simulink model "ev_tms_v4_2022"  (R2023a)
settings: Solver=VariableStepAuto  StartTime=0.0  StopTime=inf  RelTol=1e-3  AbsTol=1e-3
model workspace: external: MATLAB File /Users/rossschrader/Documents/GitHub/RL_EV_TMS/blower_control/power_comparison/ev_tms_v4_params.m (data not in the file)
undefined symbols (not defined in the file): ac_onoff, battery_C1_LUT, battery_capacity_LUT, battery_cell_cp, battery_cell_mass, battery_Em_LUT, battery_N_cells, battery_Qe_init, battery_R0_LUT, battery_R1_LUT, battery_SOC_LUT, battery_T_init, battery_temperature_LUT, bulb, cabin_duct_area, cabin_T_init, chiller_area_primary, chiller_N_baffles, chiller_N_tubes, chiller_tube_D, chiller_tube_L, chiller_wall_conductivity, chiller_wall_thickness, compressor_rpm_LUT, condenser_air_area_flow, condenser_air_area_primary, condenser_W, condenser_wall_conductivity, condenser_wall_thickness, coolant_channel_D, coolant_pipe_D, coolant_T_init, coolant_tank_area, coolant_tank_volume, coolant_valve_D_ratio_max, coolant_valve_D_ratio_min, coolant_valve_displacement, coolant_valve_S_max, evaporator_air_area_flow, evaporator_air_area_primary, evaporator_P_target, evaporator_W, evaporator_wall_conductivity, evaporator_wall_thickness, outlet, pump_speed_max, radiator_air_area_flow, radiator_air_area_primary, radiator_W, radiator_wall_conductivity, radiator_wall_thickness, refrigerant_alpha_init, refrigerant_pipe_D, T_env, T_setpoint
libraries: fl_lib x221, nesl_utility x79, SimscapeFluids_lib x25, LiBatteryElements_lib x16, sdl_lib x3, slpidlib x2, simulink x1, rllib x1, autolibshared x1, SignalEditorBlockLib x1
(part 1 of 7)
CloseFcn:
  | try,close(h1_sscfluids_ev_thermal_management),end
  | clear h1_sscfluids_ev_thermal_management
  | 
  | clear tout simlog_sscfluids_ev_thermal_management
Description:
  | Electric Vehicle Thermal Management
settings Model: Creator=The MathWorks, Inc.  LastModifiedBy=rossschrader
settings SolverCC: AutoScaleAbsTol=off  MaxConsecutiveMinStep=4  ZeroCrossAlgorithm=Adaptive  AlgebraicLoopSolver=TrustRegion  MaxZcPerStep=1
settings DebuggingCC: MaxConsecutiveZCsMsg=none  IgnoredZcDiagnostic=none  UnconnectedInputMsg=warning  UnconnectedOutputMsg=warning  UnconnectedLineMsg=warning  SymbolicDimsDataTypeCodeGenerationDiagnostic=none
settings ModelReferenceCC: EnableRefExpFcnMdlSchedulingChecks=on
settings SFSimCC: CustomCodeUndefinedFunction=UseInterfaceOnly
settings RTWCC: DLArmComputeVersion=19.05
settings SimscapeCC: SimscapeLogType=all  SimscapeLogSimulationStatistics=on  SimscapeLogName=simlog_sscfluids_ev_thermal_management  SimscapeLogDataHistory=20000

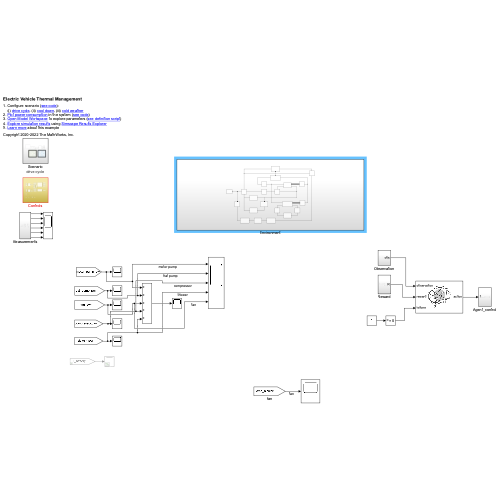
[thumbnail: Simulink's stored preview of the top-level diagram]
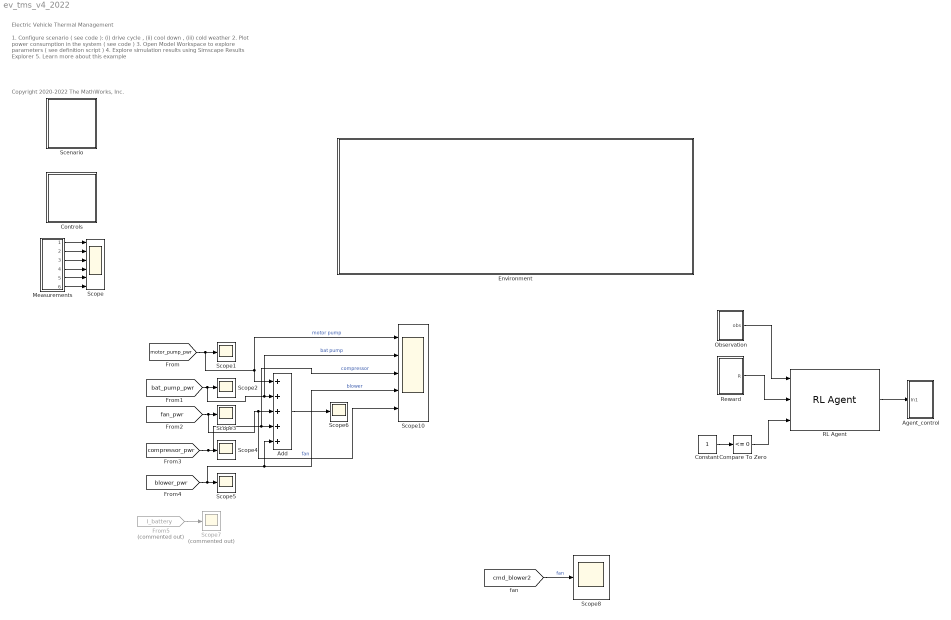
== system ev_tms_v4_2022 ==
  note: Electric Vehicle Thermal Management
  note: 1. Configure scenario ( see code ):
      | (i) drive cycle , (ii) cool down , (iii) cold weather
      | 2. Plot power consumption in the system ( see code )
      | 3. Open Model Workspace to explore parameters ( see definition script )
      | 4. Explore simulation results using Simscape Results Explorer
      | 5. Learn more about this example
  note: Copyright 2020-2022 The MathWorks, Inc.
  Add : Sum  Inputs=+++++
  Agent_control : Subsystem
  Compare To Zero : simulink/Logic and Bit Operations/Compare To Zero  relop=<=  OutDataTypeStr=boolean
  Constant : Constant
  Controls : Subsystem  Tag=PublishSubsystem
  Environment : Subsystem
  From5 : From  Commented=on  GotoTag=I_battery  TagVisibility=global
  Measurements : Subsystem
  Observation : Subsystem
  RL Agent : rllib/RL Agent  Agent=agentObj  ExternalActionAsInput=off  ProvideLastAction=off  ProvideCumRwd=off  TreatAsDirectFeedthrough=on  UseStrictObservationDataTypes=off
  Reward : Subsystem
  Scenario : Subsystem  Tag=drive cycle
      settings: AttributesFormatString=%<Tag>
  Scope : Scope  NumInputPorts=6
  Scope{1..6,8} (7 alike) : Scope
  Scope10 : Scope  NumInputPorts=5
  Scope7 : Scope  Commented=on
  wires:
  Measurements/1(Out1) -> Scope/1
  Measurements/2(Out2) -> Scope/2
  Measurements/3(Out3) -> Scope/3
  Measurements/4(Out4) -> Scope/4
  Measurements/5(Out5) -> Scope/5
  Measurements/6(Out6) -> Scope/6
  [bat_pump_pwr] -> Scope10/2, Add/2, Scope2/1  "bat pump"
  [fan_pwr] -> Scope10/5, Add/3, Scope3/1  "fan"
  [motor_pump_pwr] -> Scope10/1, Add/1, Scope1/1  "motor pump"
  [compressor_pwr] -> Scope10/3, Add/4, Scope4/1  "compressor"
  [blower_pwr] -> Scope10/4, Add/5, Scope5/1  "blower"
  Add/1 -> Scope6/1
  From5/1 -> Scope7/1
  Observation/1(obs) -> RL Agent/1
  Compare To Zero/1 -> RL Agent/3
  Constant/1 -> Compare To Zero/1
  Reward/1(R) -> RL Agent/2
  [cmd_blower2] -> Scope8/1  "fan"
  RL Agent/1 -> Agent_control/1(In1)

== system ev_tms_v4_2022/Agent_control ==
  In1 : Inport
  tag scope: cmd_blower2=global
  wires:
  In1/1 -> [cmd_blower2]

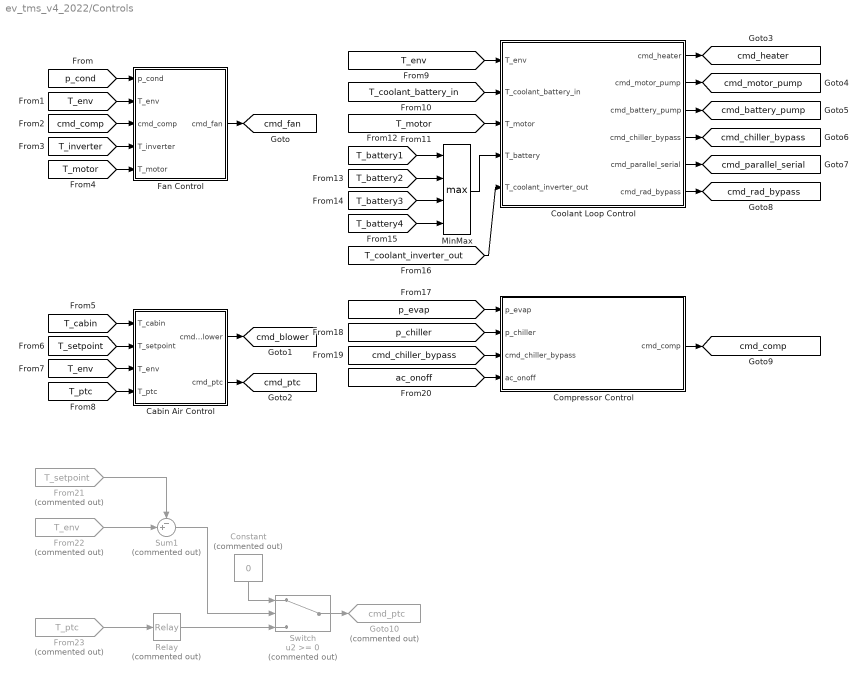
== system ev_tms_v4_2022/Controls ==
  Cabin Air Control : Subsystem
  Compressor Control : Subsystem
  Constant : Constant  Commented=on  Value=0
  Coolant Loop Control : Subsystem
  Fan Control : Subsystem
  From21 : From  Commented=on  GotoTag=T_setpoint  TagVisibility=global
  From22 : From  Commented=on  GotoTag=T_env  TagVisibility=global
  From23 : From  Commented=on  GotoTag=T_ptc  TagVisibility=global
  Goto10 : Goto  Commented=on  GotoTag=cmd_ptc  TagVisibility=global
  MinMax : MinMax  Function=max  Inputs=4
  Relay : Relay  Commented=on  OnSwitchValue=45  OffSwitchValue=35  OnOutputValue=0  OffOutputValue=1  ZeroCross=off
  Sum1 : Sum  Commented=on  Inputs=-+|
  Switch : Switch  Commented=on  SaturateOnIntegerOverflow=off  InputSameDT=off
  tag scope: cmd_battery_pump=global, cmd_blower=global, cmd_chiller_bypass=global, cmd_comp=global, cmd_fan=global, cmd_heater=global, cmd_motor_pump=global, cmd_parallel_serial=global, cmd_ptc=global, cmd_rad_bypass=global
  wires:
  [p_cond] -> Fan Control/1(p_cond)
  [T_env] -> Fan Control/2(T_env)
  [T_inverter] -> Fan Control/4(T_inverter)
  [T_motor] -> Fan Control/5(T_motor)
  [T_env] -> Coolant Loop Control/1(T_env)
  [T_coolant_battery_in] -> Coolant Loop Control/2(T_coolant_battery_in)
  Fan Control/1(cmd_fan) -> [cmd_fan]
  Coolant Loop Control/1(cmd_heater) -> [cmd_heater]
  Coolant Loop Control/2(cmd_motor_pump) -> [cmd_motor_pump]
  Coolant Loop Control/3(cmd_battery_pump) -> [cmd_battery_pump]
  [p_evap] -> Compressor Control/1(p_evap)
  [p_chiller] -> Compressor Control/2(p_chiller)
  [cmd_chiller_bypass] -> Compressor Control/3(cmd_chiller_bypass)
  [ac_onoff] -> Compressor Control/4(ac_onoff)
  Compressor Control/1(cmd_comp) -> [cmd_comp]
  Cabin Air Control/1(cmd_blower) -> [cmd_blower]
  Cabin Air Control/2(cmd_ptc) -> [cmd_ptc]
  Coolant Loop Control/4(cmd_chiller_bypass) -> [cmd_chiller_bypass]
  Coolant Loop Control/5(cmd_parallel_serial) -> [cmd_parallel_serial]
  Coolant Loop Control/6(cmd_rad_bypass) -> [cmd_rad_bypass]
  [T_motor] -> Coolant Loop Control/3(T_motor)
  [T_battery3] -> MinMax/3
  [T_battery4] -> MinMax/4
  [T_battery2] -> MinMax/2
  [T_battery1] -> MinMax/1
  [T_coolant_inverter_out] -> Coolant Loop Control/5(T_coolant_inverter_out)
  MinMax/1 -> Coolant Loop Control/4(T_battery)
  [cmd_comp] -> Fan Control/3(cmd_comp)
  [T_cabin] -> Cabin Air Control/1(T_cabin)
  [T_setpoint] -> Cabin Air Control/2(T_setpoint)
  [T_env] -> Cabin Air Control/3(T_env)
  [T_ptc] -> Cabin Air Control/4(T_ptc)
  Sum1/1 -> Switch/2
  From23/1 -> Relay/1
  Constant/1 -> Switch/1
  From21/1 -> Sum1/1
  Relay/1 -> Switch/3
  From22/1 -> Sum1/2
  Switch/1 -> Goto10/1

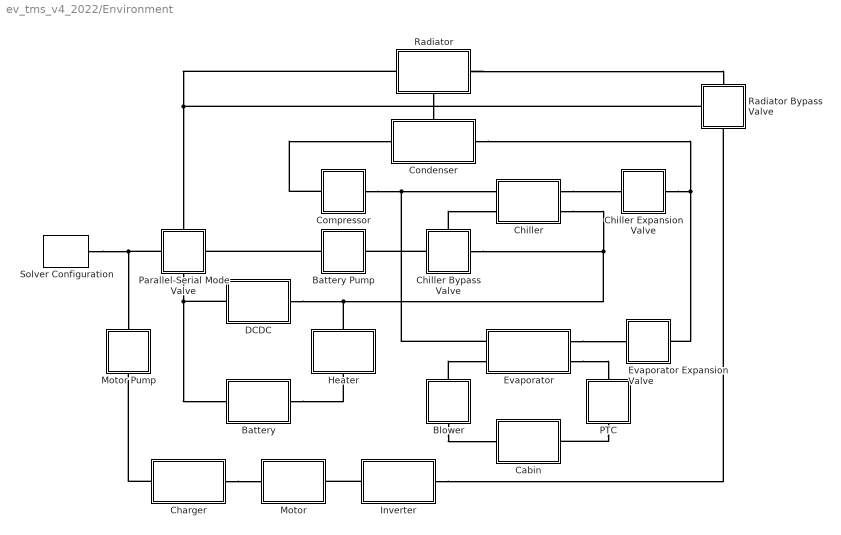
== system ev_tms_v4_2022/Environment ==
  Battery : Subsystem  Tag=PublishSubsystem
      mask Display: disp(get_param(gcb, 'Name'))
  Battery Pump : Subsystem  Tag=PublishSubsystem
      mask Display:
      | plot(100*cos(linspace(0, 2*pi, 500)), 100*sin(linspace(0, 2*pi, 500)))
      | patch([100 55 55 100]-1, [0 24 -24 0], [0 0 0])
  Blower : Subsystem  Tag=PublishSubsystem
      settings: PortSchema="{\"entries\":[{\"content\":{\"sides\":[{\"content\":{\"connectorIds\":[]},\"type\":\"ConnectorPlacement.EquallySpacedRectSide\",\"uuid\":\"e68f4e4f-d2a0-4f21-a3dd-a8ccea0ce87c\"},{\"content\":{\"connectorIds\":[],\"side\":\"RIGHT\"},\"type\":\"ConnectorPlacement.EquallySpacedRectSide\",\"uuid\":\"01f15736-e6d7-4b17-9e84-cef8e8356dfe\"},{\"content\":{\"connectorIds\":[\"LConn1\"],\"side\":\"TOP\"},\"type\":\"ConnectorPlacement.EquallySpacedRectSide\",\"uuid\":\"cb1790c7-7993-46e4-a971-f0b801f1d2ca\"},{\"content\":{\"connectorIds\":[\"RConn1\"],\"side\":\"BOTTOM\"},\"type\":\"ConnectorPlacement.EquallySpacedRectSide\",\"uuid\":\"4227c4aa-9146-4cfe-9198-d14a991805e7\"},{\"content\":{\"connectorIds\":[],\"side\":\"HIDDEN\"},\"type\":\"ConnectorPlacement.EquallySpacedRectSide\",\"uuid\":\"e2e3575c-3b20-453d-a897-62a34bc693b5\"}]},\"type\":\"ConnectorPlacement.EquallySpacedConnector\",\"uuid\":\"0a7b2bb7-4c38-48ec-bfc1-fef0f38ff266\"}],\"packageUris\":[\"http://schema.mathworks.com/mf0/Connector/R2020b\"],\"version\":\"1.0\"}"
      mask Display:
      | plot(100*cos(linspace(0, 2*pi, 500)), 100*sin(linspace(0, 2*pi, 500)))
      | plot([28 80], [96 -60])
      | plot([-28 -80], [96 -60])
      | patch(-50*sin(3*linspace(0, pi, 500)).*cos(linspace(0, pi, 500)), -50*sin(3*linspace(0, pi, 500)).*sin(linspace(0, pi, 500)), [0 0 0])
  Cabin : Subsystem  Tag=PublishSubsystem
      mask Display: disp(get_param(gcb, 'Name'))
  Charger : Subsystem  Tag=PublishSubsystem
      mask Display: disp(get_param(gcb, 'Name'))
  Chiller : Subsystem  Tag=PublishSubsystem
      mask Display: disp(get_param(gcb, 'Name'))
  Chiller Bypass Valve : Subsystem  Tag=PublishSubsystem
      settings: PortSchema="{\"entries\":[{\"content\":{\"sides\":[{\"content\":{\"connectorIds\":[\"LConn1\"]},\"type\":\"ConnectorPlacement.EquallySpacedRectSide\",\"uuid\":\"c08eba77-a229-49ef-96a6-5debb89bda6a\"},{\"content\":{\"connectorIds\":[\"RConn1\"],\"side\":\"RIGHT\"},\"type\":\"ConnectorPlacement.EquallySpacedRectSide\",\"uuid\":\"bf1c3c92-2d76-498b-aaec-772d925127f1\"},{\"content\":{\"connectorIds\":[\"LConn2\"],\"side\":\"TOP\"},\"type\":\"ConnectorPlacement.EquallySpacedRectSide\",\"uuid\":\"93e37f17-addf-4d5b-9a57-68c15f6f3e9e\"},{\"content\":{\"connectorIds\":[],\"side\":\"HIDDEN\"},\"type\":\"ConnectorPlacement.EquallySpacedRectSide\",\"uuid\":\"04fa26e7-4471-4f20-81b8-29848726d0cd\"}]},\"type\":\"ConnectorPlacement.EquallySpacedConnector\",\"uuid\":\"712c9662-e870-49a5-b0e3-dc86b008bacd\"}],\"packageUris\":[\"http://schema.mathworks.com/mf0/Connector/R2020b\"],\"version\":\"1.0\"}"
      mask Display:
      | color('white')
      | plot(100, 100)
      | plot(-100, -100)
      | color('black')
      | 
      | plot([0 -100 -100 0], [0 50 -50 0])
      | plot([0 100 100 0], [0 50 -50 0])
      | plot([0 50 -50 0], [0 100 100 0])
  Chiller Expansion Valve : Subsystem  Tag=PublishSubsystem
      mask Display:
      | color('white')
      | plot(100, 100)
      | plot(-100, -100)
      | color('black')
      | 
      | plot([0 -100 -100 0], [0 50 -50 0])
      | plot([0 100 100 0], [0 50 -50 0])
  Compressor : Subsystem  Tag=PublishSubsystem
      mask Display:
      | plot(100*cos(linspace(0, 2*pi, 500)), 100*sin(linspace(0, 2*pi, 500)))
      | plot([-96 60], [28 80])
      | plot([-96 60], [-28 -80])
  Condenser : Subsystem  Tag=PublishSubsystem
      settings: PortSchema="{\"entries\":[{\"content\":{\"sides\":[{\"content\":{\"connectorIds\":[\"LConn1\"]},\"type\":\"ConnectorPlacement.EquallySpacedRectSide\",\"uuid\":\"1c8aa983-a374-4f1b-b303-31d972477bc1\"},{\"content\":{\"connectorIds\":[\"RConn1\"],\"side\":\"RIGHT\"},\"type\":\"ConnectorPlacement.EquallySpacedRectSide\",\"uuid\":\"9470a7c4-8d01-4f33-b281-130c1633b9af\"},{\"content\":{\"connectorIds\":[\"LConn2\"],\"side\":\"TOP\"},\"type\":\"ConnectorPlacement.EquallySpacedRectSide\",\"uuid\":\"521bcd61-502e-4408-add3-862bd83fd72a\"},{\"content\":{\"connectorIds\":[],\"side\":\"HIDDEN\"},\"type\":\"ConnectorPlacement.EquallySpacedRectSide\",\"uuid\":\"1fd51896-89cd-4b86-8982-5d9c8888072c\"}]},\"type\":\"ConnectorPlacement.EquallySpacedConnector\",\"uuid\":\"d9db812f-15c4-4875-aa5b-4de8fb002b03\"}],\"packageUris\":[\"http://schema.mathworks.com/mf0/Connector/R2020b\"],\"version\":\"1.0\"}"
      mask Display: disp(get_param(gcb, 'Name'))
  DCDC : Subsystem  Tag=PublishSubsystem
      mask Display: disp(get_param(gcb, 'Name'))
  Evaporator : Subsystem  Tag=PublishSubsystem
      mask Display: disp(get_param(gcb, 'Name'))
  Evaporator Expansion Valve : Subsystem  Tag=PublishSubsystem
      mask Display:
      | color('white')
      | plot(100, 100)
      | plot(-100, -100)
      | color('black')
      | 
      | plot([0 -100 -100 0], [0 50 -50 0])
      | plot([0 100 100 0], [0 50 -50 0])
  Heater : Subsystem  Tag=PublishSubsystem
      settings: PortSchema="{\"entries\":[{\"content\":{\"sides\":[{\"content\":{\"connectorIds\":[]},\"type\":\"ConnectorPlacement.EquallySpacedRectSide\",\"uuid\":\"e68f4e4f-d2a0-4f21-a3dd-a8ccea0ce87c\"},{\"content\":{\"connectorIds\":[],\"side\":\"RIGHT\"},\"type\":\"ConnectorPlacement.EquallySpacedRectSide\",\"uuid\":\"01f15736-e6d7-4b17-9e84-cef8e8356dfe\"},{\"content\":{\"connectorIds\":[\"LConn1\"],\"side\":\"TOP\"},\"type\":\"ConnectorPlacement.EquallySpacedRectSide\",\"uuid\":\"cb1790c7-7993-46e4-a971-f0b801f1d2ca\"},{\"content\":{\"connectorIds\":[\"RConn1\"],\"side\":\"BOTTOM\"},\"type\":\"ConnectorPlacement.EquallySpacedRectSide\",\"uuid\":\"c273a181-4a30-4811-b574-293af963aa70\"},{\"content\":{\"connectorIds\":[],\"side\":\"HIDDEN\"},\"type\":\"ConnectorPlacement.EquallySpacedRectSide\",\"uuid\":\"e2e3575c-3b20-453d-a897-62a34bc693b5\"}]},\"type\":\"ConnectorPlacement.EquallySpacedConnector\",\"uuid\":\"0a7b2bb7-4c38-48ec-bfc1-fef0f38ff266\"}],\"packageUris\":[\"http://schema.mathworks.com/mf0/Connector/R2020b\"],\"version\":\"1.0\"}"
      mask Display: disp(get_param(gcb, 'Name'))
  Inverter : Subsystem  Tag=PublishSubsystem
      mask Display: disp(get_param(gcb, 'Name'))
  Motor : Subsystem  Tag=PublishSubsystem
      mask Display: disp(get_param(gcb, 'Name'))
  Motor Pump : Subsystem  Tag=PublishSubsystem
      settings: PortSchema="{\"entries\":[{\"content\":{\"sides\":[{\"content\":{\"connectorIds\":[]},\"type\":\"ConnectorPlacement.EquallySpacedRectSide\",\"uuid\":\"e68f4e4f-d2a0-4f21-a3dd-a8ccea0ce87c\"},{\"content\":{\"connectorIds\":[],\"side\":\"RIGHT\"},\"type\":\"ConnectorPlacement.EquallySpacedRectSide\",\"uuid\":\"01f15736-e6d7-4b17-9e84-cef8e8356dfe\"},{\"content\":{\"connectorIds\":[\"LConn1\"],\"side\":\"TOP\"},\"type\":\"ConnectorPlacement.EquallySpacedRectSide\",\"uuid\":\"cb1790c7-7993-46e4-a971-f0b801f1d2ca\"},{\"content\":{\"connectorIds\":[\"RConn1\"],\"side\":\"BOTTOM\"},\"type\":\"ConnectorPlacement.EquallySpacedRectSide\",\"uuid\":\"8246d38e-a008-4f4a-9c4c-9e03a2298f65\"},{\"content\":{\"connectorIds\":[],\"side\":\"HIDDEN\"},\"type\":\"ConnectorPlacement.EquallySpacedRectSide\",\"uuid\":\"e2e3575c-3b20-453d-a897-62a34bc693b5\"}]},\"type\":\"ConnectorPlacement.EquallySpacedConnector\",\"uuid\":\"0a7b2bb7-4c38-48ec-bfc1-fef0f38ff266\"}],\"packageUris\":[\"http://schema.mathworks.com/mf0/Connector/R2020b\"],\"version\":\"1.0\"}"
      mask Display:
      | plot(100*cos(linspace(0, 2*pi, 500)), 100*sin(linspace(0, 2*pi, 500)))
      | patch([0 24 -24 0], [-100 -55 -55 -100]+1, [0 0 0])
  PTC : Subsystem  Tag=PublishSubsystem
      settings: PortSchema="{\"entries\":[{\"content\":{\"sides\":[{\"content\":{\"connectorIds\":[]},\"type\":\"ConnectorPlacement.EquallySpacedRectSide\",\"uuid\":\"e68f4e4f-d2a0-4f21-a3dd-a8ccea0ce87c\"},{\"content\":{\"connectorIds\":[],\"side\":\"RIGHT\"},\"type\":\"ConnectorPlacement.EquallySpacedRectSide\",\"uuid\":\"01f15736-e6d7-4b17-9e84-cef8e8356dfe\"},{\"content\":{\"connectorIds\":[\"LConn1\"],\"side\":\"TOP\"},\"type\":\"ConnectorPlacement.EquallySpacedRectSide\",\"uuid\":\"cb1790c7-7993-46e4-a971-f0b801f1d2ca\"},{\"content\":{\"connectorIds\":[\"RConn1\"],\"side\":\"BOTTOM\"},\"type\":\"ConnectorPlacement.EquallySpacedRectSide\",\"uuid\":\"8429c419-0ca8-47a9-96c7-e8d1ee01deb6\"},{\"content\":{\"connectorIds\":[],\"side\":\"HIDDEN\"},\"type\":\"ConnectorPlacement.EquallySpacedRectSide\",\"uuid\":\"e2e3575c-3b20-453d-a897-62a34bc693b5\"}]},\"type\":\"ConnectorPlacement.EquallySpacedConnector\",\"uuid\":\"0a7b2bb7-4c38-48ec-bfc1-fef0f38ff266\"}],\"packageUris\":[\"http://schema.mathworks.com/mf0/Connector/R2020b\"],\"version\":\"1.0\"}"
      mask Display: disp(get_param(gcb, 'Name'))
  Parallel-Serial Mode Valve : Subsystem  Tag=PublishSubsystem
      settings: PortSchema="{\"entries\":[{\"content\":{\"sides\":[{\"content\":{\"connectorIds\":[\"LConn1\"]},\"type\":\"ConnectorPlacement.EquallySpacedRectSide\",\"uuid\":\"769cdae0-dc58-4cfd-92d9-ac32508c6b10\"},{\"content\":{\"connectorIds\":[\"RConn1\"],\"side\":\"RIGHT\"},\"type\":\"ConnectorPlacement.EquallySpacedRectSide\",\"uuid\":\"df63fb06-baf4-4717-a479-9d23ab47f4aa\"},{\"content\":{\"connectorIds\":[\"LConn2\"],\"side\":\"TOP\"},\"type\":\"ConnectorPlacement.EquallySpacedRectSide\",\"uuid\":\"82fb49eb-ec90-48c3-a5a6-67a52560ca4a\"},{\"content\":{\"connectorIds\":[\"RConn2\"],\"side\":\"BOTTOM\"},\"type\":\"ConnectorPlacement.EquallySpacedRectSide\",\"uuid\":\"ab7ba56f-69df-4d32-95cc-f479df491f70\"},{\"content\":{\"connectorIds\":[],\"side\":\"HIDDEN\"},\"type\":\"ConnectorPlacement.EquallySpacedRectSide\",\"uuid\":\"14514675-c4ca-4da0-9eea-4f242d50599f\"}]},\"type\":\"ConnectorPlacement.EquallySpacedConnector\",\"uuid\":\"38d91077-2bde-4773-8967-83aa2a8f4957\"}],\"packageUris\":[\"http://schema.mathworks.com/mf0/Connector/R2020b\"],\"version\":\"1.0\"}"
      mask Display:
      | color('white')
      | plot(100, 100)
      | plot(-100, -100)
      | color('black')
      | 
      | plot([0 -100 -100 0], [0 50 -50 0])
      | plot([0 100 100 0], [0 50 -50 0])
      | plot([0 50 -50 0], [0 100 100 0])
      | plot([0 50 -50 0], [0 -100 -100 0])
  Radiator : Subsystem  Tag=PublishSubsystem
      settings: PortSchema="{\"entries\":[{\"content\":{\"sides\":[{\"content\":{\"connectorIds\":[\"LConn1\"]},\"type\":\"ConnectorPlacement.EquallySpacedRectSide\",\"uuid\":\"c41edd26-4d41-4ef4-bf36-0d7d2de0fe84\"},{\"content\":{\"connectorIds\":[\"RConn1\"],\"side\":\"RIGHT\"},\"type\":\"ConnectorPlacement.EquallySpacedRectSide\",\"uuid\":\"d74127b5-b0c6-43ff-8d29-bbb0795bdd4e\"},{\"content\":{\"connectorIds\":[],\"side\":\"TOP\"},\"type\":\"ConnectorPlacement.EquallySpacedRectSide\",\"uuid\":\"8924700c-666b-431d-af64-838d19a43fe5\"},{\"content\":{\"connectorIds\":[\"RConn2\"],\"side\":\"BOTTOM\"},\"type\":\"ConnectorPlacement.EquallySpacedRectSide\",\"uuid\":\"806c213f-7f35-4ea6-bb4b-65a47516f414\"},{\"content\":{\"connectorIds\":[],\"side\":\"HIDDEN\"},\"type\":\"ConnectorPlacement.EquallySpacedRectSide\",\"uuid\":\"7380b933-a71f-43b9-ae5a-a995a710e36b\"}]},\"type\":\"ConnectorPlacement.EquallySpacedConnector\",\"uuid\":\"07da1dfa-e3e5-4e48-89d5-0544451f2413\"}],\"packageUris\":[\"http://schema.mathworks.com/mf0/Connector/R2020b\"],\"version\":\"1.0\"}"
      mask Display: disp(get_param(gcb, 'Name'))
  Radiator Bypass Valve : Subsystem  Tag=PublishSubsystem
      settings: PortSchema="{\"entries\":[{\"content\":{\"sides\":[{\"content\":{\"connectorIds\":[\"LConn1\"]},\"type\":\"ConnectorPlacement.EquallySpacedRectSide\",\"uuid\":\"1991dfbd-c304-4807-b100-246bfad34882\"},{\"content\":{\"connectorIds\":[],\"side\":\"RIGHT\"},\"type\":\"ConnectorPlacement.EquallySpacedRectSide\",\"uuid\":\"8dd83d3e-3811-40e7-af6b-04929d024ef5\"},{\"content\":{\"connectorIds\":[\"LConn2\"],\"side\":\"TOP\"},\"type\":\"ConnectorPlacement.EquallySpacedRectSide\",\"uuid\":\"fac05c8b-fd4c-4caf-8f39-67a22531bfff\"},{\"content\":{\"connectorIds\":[\"RConn1\"],\"side\":\"BOTTOM\"},\"type\":\"ConnectorPlacement.EquallySpacedRectSide\",\"uuid\":\"fc2a2150-414c-4914-a21f-f7fbe52b92e3\"},{\"content\":{\"connectorIds\":[],\"side\":\"HIDDEN\"},\"type\":\"ConnectorPlacement.EquallySpacedRectSide\",\"uuid\":\"26904e98-8b18-4b4d-8057-298167e4cabd\"}]},\"type\":\"ConnectorPlacement.EquallySpacedConnector\",\"uuid\":\"c94d3059-f972-4f57-b434-9a5f1e7a2893\"}],\"packageUris\":[\"http://schema.mathworks.com/mf0/Connector/R2020b\"],\"version\":\"1.0\"}"
      mask Display:
      | color('white')
      | plot(100, 100)
      | plot(-100, -100)
      | color('black')
      | 
      | plot([0 -100 -100 0], [0 50 -50 0])
      | plot([0 50 -50 0], [0 100 100 0])
      | plot([0 50 -50 0], [0 -100 -100 0])
  Solver Configuration : nesl_utility/Solver Configuration  PhysicalDomain=network_engine_domain  SubClassName=solver  LeftPortType=input  RightPortType=generic  Tones=[]  Harmonics=[]  SimulateNoise=off  Profile=off  UseLocalSampling=off  EnableSwitchedLinearOptims=on  FrequencyDomain=off  UseCCode=off  RelTol=0.001  AbsTol=1e-06  MinStep=1e-09  ToWorkspace=off  RevertToSquareIcSolve=off  NumHomotopyIterations=100  PhasorMode=off  PhasorModeNumHarmonics=1  ConsistencySolver=NEWTON_XTOL_AFTER_FTOL  IndexReductionMethod=DerivativeReplacement  DoDC=off  ResidualTolerance=1e-09  ConsistencyTolSource=GLOBAL  ConsistencyAbsTol=0.001  ConsistencyRelTol=0.001  ConsistencyTolFactor=0.001  UseLocalSolver=off  LocalSolverChoice=NE_BACKWARD_EULER_ADVANCER  ResolveIndetEquations=on  FunctionEvalNumThread=1  LocalSolverSampleTime=0.001  DoFixedCost=off  MaxNonlinIter=3  MaxModeIter=2  ComputeImpulses=off  ImpulseIterations=2  LinearAlgebra=auto  LinearAlgebraNumThread=0  EquationFormulation=NE_TIME_EF  DelaysMemoryBudget=1024  AutomaticFiltering=on  FilteringTimeConstant=0.001  PartitionStorageMethod=AS_NEEDED  PartitionMemoryBudget=1024  PartitionMethod=ROBUST
  connections:
  Inverter/RConn1 -- Radiator Bypass Valve/RConn1
  Evaporator/RConn2 -- PTC/LConn1
  Parallel-Serial Mode Valve/LConn1 -- Solver Configuration/RConn1 -- Motor Pump/LConn1
  PTC/RConn1 -- Cabin/RConn1
  Blower/LConn1 -- Evaporator/LConn2
  Blower/RConn1 -- Cabin/LConn1
  Condenser/RConn1 -- Chiller Expansion Valve/RConn1 -- Evaporator Expansion Valve/RConn1
  Radiator/RConn1 -- Radiator Bypass Valve/LConn2
  Evaporator/RConn1 -- Evaporator Expansion Valve/LConn1
  Battery/RConn1 -- Heater/RConn1
  Chiller Bypass Valve/LConn1 -- Battery Pump/RConn1
  Radiator/RConn2 -- Condenser/LConn2
  Radiator/LConn1 -- Radiator Bypass Valve/LConn1 -- Parallel-Serial Mode Valve/LConn2
  Compressor/RConn1 -- Evaporator/LConn1 -- Chiller/LConn1
  Parallel-Serial Mode Valve/RConn2 -- DCDC/LConn1 -- Battery/LConn1
  Charger/RConn1 -- Motor/LConn1
  Chiller/RConn2 -- DCDC/RConn1 -- Heater/LConn1 -- Chiller Bypass Valve/RConn1
  Charger/LConn1 -- Motor Pump/RConn1
  Battery Pump/LConn1 -- Parallel-Serial Mode Valve/RConn1
  Chiller/RConn1 -- Chiller Expansion Valve/LConn1
  Chiller Bypass Valve/LConn2 -- Chiller/LConn2
  Compressor/LConn1 -- Condenser/LConn1
  Inverter/LConn1 -- Motor/RConn1

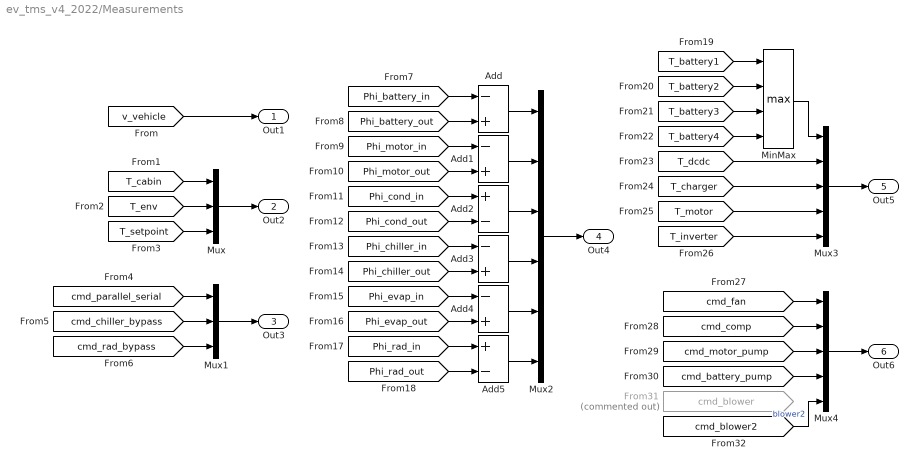
== system ev_tms_v4_2022/Measurements ==
  Add{,1,3..4} (4 alike) : Sum  Inputs=-+
  Add2 : Sum  Inputs=+-
  Add5 : Sum  Inputs=+-
  From31 : From  Commented=on  GotoTag=cmd_blower  TagVisibility=global
  MinMax : MinMax  Function=max  Inputs=4
  Mux : Mux  Inputs=3
  Mux1 : Mux  Inputs=3
  Mux2 : Mux  Inputs=6
  Mux3 : Mux  Inputs=5
  Mux4 : Mux  Inputs=5
  Out1 : Outport
  Out2 : Outport  Port=2
  Out3 : Outport  Port=3
  Out4 : Outport  Port=4
  Out5 : Outport  Port=5
  Out6 : Outport  Port=6
  wires:
  [v_vehicle] -> Out1/1
  [T_cabin] -> Mux/1
  [T_env] -> Mux/2
  [T_setpoint] -> Mux/3
  Mux/1 -> Out2/1
  [cmd_parallel_serial] -> Mux1/1
  [cmd_chiller_bypass] -> Mux1/2
  [cmd_rad_bypass] -> Mux1/3
  Mux1/1 -> Out3/1
  [Phi_battery_in] -> Add/1
  [Phi_battery_out] -> Add/2
  [Phi_motor_in] -> Add1/1
  [Phi_motor_out] -> Add1/2
  [Phi_cond_in] -> Add2/1
  [Phi_cond_out] -> Add2/2
  [Phi_chiller_in] -> Add3/1
  [Phi_chiller_out] -> Add3/2
  [Phi_evap_in] -> Add4/1
  [Phi_evap_out] -> Add4/2
  [Phi_rad_in] -> Add5/1
  [Phi_rad_out] -> Add5/2
  Add/1 -> Mux2/1
  Add1/1 -> Mux2/2
  Add2/1 -> Mux2/3
  Add3/1 -> Mux2/4
  Add4/1 -> Mux2/5
  Add5/1 -> Mux2/6
  Mux2/1 -> Out4/1
  [T_battery1] -> MinMax/1
  [T_battery2] -> MinMax/2
  [T_battery3] -> MinMax/3
  [T_battery4] -> MinMax/4
  [T_dcdc] -> Mux3/2
  [T_charger] -> Mux3/3
  [T_motor] -> Mux3/4
  [T_inverter] -> Mux3/5
  MinMax/1 -> Mux3/1
  Mux3/1 -> Out5/1
  [cmd_fan] -> Mux4/1
  [cmd_comp] -> Mux4/2
  [cmd_motor_pump] -> Mux4/3
  [cmd_battery_pump] -> Mux4/4
  Mux4/1 -> Out6/1
  [cmd_blower2] -> Mux4/5  "blower2"

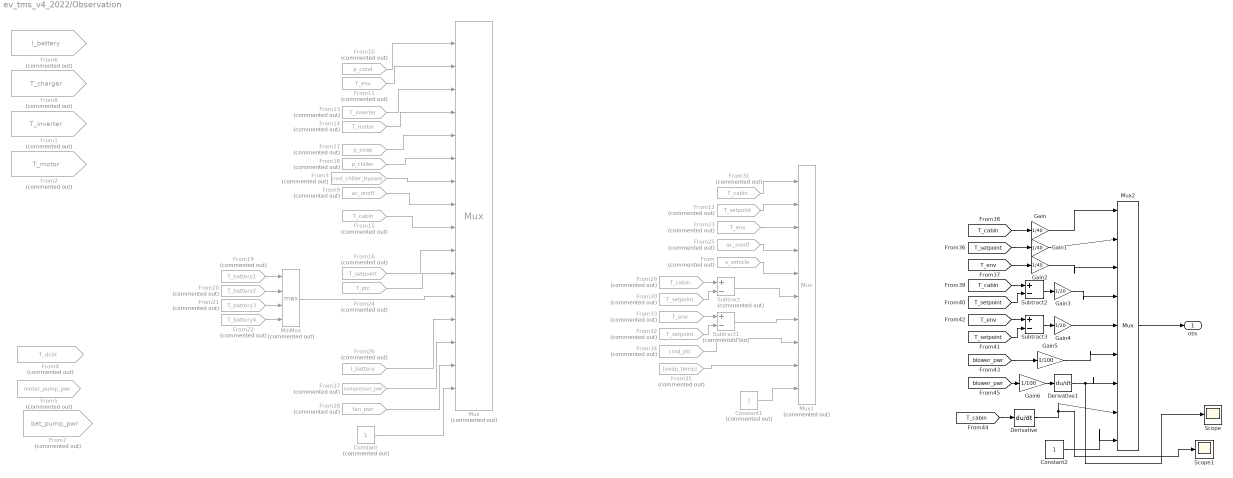
== system ev_tms_v4_2022/Observation ==
  Constant : Constant  Commented=on
  Constant1 : Constant  Commented=on
  Constant2 : Constant
  Derivative : Derivative
  Derivative1 : Derivative
  From : From  Commented=on  GotoTag=v_vehicle  TagVisibility=global
  From1 : From  Commented=on  GotoTag=T_inverter  TagVisibility=global
  From10 : From  Commented=on  GotoTag=p_cond  TagVisibility=global
  From11 : From  Commented=on  GotoTag=T_env  TagVisibility=global
  From{12,16,30,32} (4 alike) : From  Commented=on  GotoTag=T_setpoint  TagVisibility=global
  From13 : From  Commented=on  GotoTag=T_inverter  TagVisibility=global
  From14 : From  Commented=on  GotoTag=T_motor  TagVisibility=global
  From15 : From  Commented=on  GotoTag=T_cabin  TagVisibility=global
  From17 : From  Commented=on  GotoTag=p_evap  TagVisibility=global
  From18 : From  Commented=on  GotoTag=p_chiller  TagVisibility=global
  From19 : From  Commented=on  GotoTag=T_battery1  TagVisibility=global
  From2 : From  Commented=on  GotoTag=T_motor  TagVisibility=global
  From20 : From  Commented=on  GotoTag=T_battery2  TagVisibility=global
  From21 : From  Commented=on  GotoTag=T_battery3  TagVisibility=global
  From22 : From  Commented=on  GotoTag=T_battery4  TagVisibility=global
  From23 : From  Commented=on  GotoTag=T_env  TagVisibility=global
  From24 : From  Commented=on  GotoTag=T_ptc  TagVisibility=global
  From25 : From  Commented=on  GotoTag=ac_onoff  TagVisibility=global
  From26 : From  Commented=on  GotoTag=I_battery  TagVisibility=global
  From27 : From  Commented=on  GotoTag=compressor_pwr  TagVisibility=global
  From28 : From  Commented=on  GotoTag=fan_pwr  TagVisibility=global
  From29 : From  Commented=on  GotoTag=T_cabin  TagVisibility=global
  From3 : From  Commented=on  GotoTag=cmd_chiller_bypass  TagVisibility=global
  From31 : From  Commented=on  GotoTag=T_cabin  TagVisibility=global
  From33 : From  Commented=on  GotoTag=T_env  TagVisibility=global
  From34 : From  Commented=on  GotoTag=cmd_ptc  TagVisibility=global
  From35 : From  Commented=on  GotoTag=evap_temp  TagVisibility=global
  From4 : From  Commented=on  GotoTag=T_dcdc  TagVisibility=global
  From5 : From  Commented=on  GotoTag=motor_pump_pwr  TagVisibility=global
  From6 : From  Commented=on  GotoTag=I_battery  TagVisibility=global
  From7 : From  Commented=on  GotoTag=bat_pump_pwr  TagVisibility=global
  From8 : From  Commented=on  GotoTag=T_charger  TagVisibility=global
  From9 : From  Commented=on  GotoTag=ac_onoff  TagVisibility=global
  Gain : Gain  Gain=1/40
  Gain1 : Gain  Gain=1/40
  Gain2 : Gain  Gain=1/40
  Gain3 : Gain  Gain=1/20
  Gain4 : Gain  Gain=1/20
  Gain5 : Gain  Gain=1/100
  Gain6 : Gain  Gain=1/100
  MinMax : MinMax  Commented=on  Function=max  Inputs=4
  Mux : Mux  Commented=on  Inputs=16
  Mux1 : Mux  Commented=on  Inputs=10
  Mux2 : Mux  Inputs=9
  Scope : Scope
  Scope1 : Scope
  Subtract : Sum  Commented=on  Inputs=+-
  Subtract1 : Sum  Commented=on  Inputs=+-
  Subtract2 : Sum  Inputs=+-
  Subtract3 : Sum  Inputs=+-
  obs : Outport
  wires:
  From19/1 -> MinMax/1
  From20/1 -> MinMax/2
  From22/1 -> MinMax/4
  From21/1 -> MinMax/3
  MinMax/1 -> Mux/12
  From10/1 -> Mux/1
  From11/1 -> Mux/2
  From13/1 -> Mux/3
  From14/1 -> Mux/4
  From17/1 -> Mux/5
  From18/1 -> Mux/6
  From3/1 -> Mux/7
  From9/1 -> Mux/8
  From15/1 -> Mux/9
  From16/1 -> Mux/10
  From24/1 -> Mux/11
  From26/1 -> Mux/13
  From27/1 -> Mux/14
  From28/1 -> Mux/15
  Constant/1 -> Mux/16
  From31/1 -> Mux1/1
  From12/1 -> Mux1/2
  From23/1 -> Mux1/3
  From25/1 -> Mux1/4
  From/1 -> Mux1/5
  Constant1/1 -> Mux1/10
  From29/1 -> Subtract/1
  From30/1 -> Subtract/2
  Subtract/1 -> Mux1/6
  From33/1 -> Subtract1/1
  From32/1 -> Subtract1/2
  Subtract1/1 -> Mux1/7
  From34/1 -> Mux1/8
  From35/1 -> Mux1/9
  [T_cabin] -> Subtract2/1
  [T_env] -> Subtract3/1
  [T_setpoint] -> Subtract2/2
  [T_setpoint] -> Subtract3/2
  Mux2/1 -> obs/1
  [T_cabin] -> Gain/1
  [T_setpoint] -> Gain1/1
  [T_env] -> Gain2/1
  Subtract2/1 -> Gain3/1
  Subtract3/1 -> Gain4/1
  [blower_pwr] -> Gain5/1
  Gain/1 -> Mux2/1
  Gain1/1 -> Mux2/2
  Gain2/1 -> Mux2/3
  Gain3/1 -> Mux2/4
  Gain4/1 -> Mux2/5
  Gain5/1 -> Mux2/6
  Constant2/1 -> Mux2/9
  [T_cabin] -> Derivative/1
  Derivative/1 -> Scope1/1, Mux2/8
  [blower_pwr] -> Gain6/1
  Gain6/1 -> Derivative1/1
  Derivative1/1 -> Scope/1, Mux2/7

== system ev_tms_v4_2022/Reward ==
  Add : Sum
  Power Reward : Subsystem
  Scope : Scope  NumInputPorts=2
  Temp Reward : Subsystem
  R : Outport
  wires:
  Add/1 -> R/1
  Power Reward/1(Power) -> Scope/1, Add/1
  Temp Reward/1(Temp) -> Scope/2, Add/2

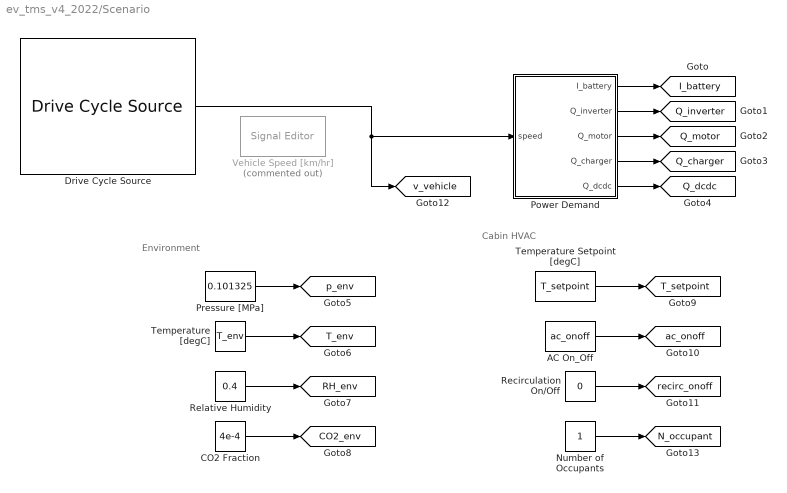
== system ev_tms_v4_2022/Scenario ==
  note: Environment
  note: Cabin HVAC
  AC On_Off : Constant  Value=ac_onoff
  CO2 Fraction : Constant  Value=4e-4
  Drive Cycle Source : autolibshared/Drive Cycle Source  cycleVar=US06  fileVar=cycleFTP75.mat  tfinal="600  seconds"  cycleRepeat=off  outAccPort=off  outGearPort=off  gearList=No gear data  t_wot1=5  xdot_woto=0  xdot_wot1=30  t_wot2=20  xdot_wot2=0  t_wotend=30  srcUnit=m/s  outUnit=km/hr  srcAccUnit=m/s/s  outAccUnit=m/s^2  dt=0  aMode=1  faultOption=off  velBnd=2  velBndUnit=mph  inUnit=m/s  timeBnd=1  failOption=off  stopSim=off  maxFaultCnt=10  maxFaultTime=2  maxTotFaultTime=15  traceOption=off  dtTrace=1  traceWindow=10  lastDCname=US06  lastOutUnit=mph  lastDT=0  lastTB=1  lastSB=2  forceCalcBound=off
  Number of Occupants : Constant
  Power Demand : Subsystem
  Pressure [MPa] : Constant  Value=0.101325
  Recirculation On/Off : Constant  Value=0
  Relative Humidity : Constant  Value=0.4
  Temperature Setpoint [degC] : Constant  Value=T_setpoint
  Temperature [degC] : Constant  Value=T_env
  Vehicle Speed [km/hr] : SignalEditorBlockLib/Signal Editor  Commented=on  FileName=sscfluids_ev_thermal_management.mat  ActiveScenario=Drive_Cycle  ActiveSignal=speed  IsBus=off  OutputBusObjectStr=Bus: BusObject  SampleTime=0  ZeroCross=off  OutputAfterFinalValue=Extrapolation  Unit=inherit  PreserveSignalName=on  ApplySigPropsToAllScenarios=on
  tag scope: CO2_env=global, I_battery=global, N_occupant=global, Q_charger=global, Q_dcdc=global, Q_inverter=global, Q_motor=global, RH_env=global, T_env=global, T_setpoint=global, ac_onoff=global, p_env=global, recirc_onoff=global, v_vehicle=global
  wires:
  Pressure [MPa]/1 -> [p_env]
  Temperature [degC]/1 -> [T_env]
  CO2 Fraction/1 -> [CO2_env]
  Temperature Setpoint [degC]/1 -> [T_setpoint]
  AC On_Off/1 -> [ac_onoff]
  Recirculation On/Off/1 -> [recirc_onoff]
  Relative Humidity/1 -> [RH_env]
  Power Demand/1(I_battery) -> [I_battery]
  Power Demand/2(Q_inverter) -> [Q_inverter]
  Power Demand/3(Q_motor) -> [Q_motor]
  Power Demand/4(Q_charger) -> [Q_charger]
  Power Demand/5(Q_dcdc) -> [Q_dcdc]
  Number of Occupants/1 -> [N_occupant]
  Drive Cycle Source/1 -> Power Demand/1(speed), [v_vehicle]

== system ev_tms_v4_2022/Controls/Cabin Air Control ==
  T_cabin : Inport
  T_setpoint : Inport  Port=2
  T_env : Inport  Port=3
  T_ptc : Inport  Port=4
  Constant : Constant  Value=0
  PID Controller : slpidlib/PID Controller  Controller=PI  Form=Ideal  TimeDomain=Continuous-time  UseExternalTs=off  SampleTime=-1  IntegratorMethod=Forward Euler  FilterMethod=Forward Euler  ControllerParametersSource=internal  P=1/50  I=1/150  UseKiTs=off  D=0  N=100  UseFilter=on  TunerSelectOption=Transfer Function Based (PID Tuner App)  InitialConditionSource=internal  InitialConditionForIntegrator=0  InitialConditionForFilter=0  DifferentiatorICPrevScaledInput=0  ExternalReset=none  TrackingMode=off  Kt=1  LimitOutput=on  SatLimitsSource=internal  UpperSaturationLimit=1  LowerSaturationLimit=0  LinearizeAsGain=on  AntiWindupMode=back-calculation  Kb=1  LimitIntegrator=off  UpperIntegratorSaturationLimit=inf  LowerIntegratorSaturationLimit=-inf  POutMin=[]  POutMax=[]  IOutMin=[]  IOutMax=[]  DOutMin=[]  DOutMax=[]  NOutMin=[]  NOutMax=[]  SumOutMin=[]  SumOutMax=[]  SaturationOutMin=[]  SaturationOutMax=[]  PParamMin=[]  PParamMax=[]  IParamMin=[]  IParamMax=[]  DParamMin=[]  DParamMax=[]  NParamMin=[]  NParamMax=[]  KbParamMin=[]  KbParamMax=[]  KtParamMin=[]  KtParamMax=[]  KbOutMin=[]  KbOutMax=[]  KtOutMin=[]  KtOutMax=[]  IntegratorOutMin=[]  IntegratorOutMax=[]  FilterOutMin=[]  FilterOutMax=[]  SumI1OutMin=[]  SumI1OutMax=[]  SumI2OutMin=[]  SumI2OutMax=[]  SumI3OutMin=[]  SumI3OutMax=[]  SumI4OutMin=[]  SumI4OutMax=[]  SumDOutMin=[]  SumDOutMax=[]  DifferentiatorOutMin=[]  DifferentiatorOutMax=[]  FilterDiffOutCoefMin=[]  FilterDiffOutCoefMax=[]  ReciprocalOutMin=[]  ReciprocalOutMax=[]  SumDenOutMin=[]  SumDenOutMax=[]  SumNumOutMin=[]  SumNumOutMax=[]  DivideOutMin=[]  DivideOutMax=[]  UdiffTsProdOutMin=[]  UdiffTsProdOutMax=[]  NTsProdOutMin=[]  NTsProdOutMax=[]  UintegralTsProdOutMin=[]  UintegralTsProdOutMax=[]  UngainTsProdOutMin=[]  UngainTsProdOutMax=[]  ClampingZeroOutDataTypeStr=Inherit: Inherit via back propagation  ClampingZeroOutMin=[]  ClampingZeroOutMax=[]  FilterDenConstantOutDataTypeStr=Inherit: Inherit via back propagation  FilterDenConstantOutMin=[]  FilterDenConstantOutMax=[]  PCopyOutDataTypeStr=Inherit: Inherit via back propagation  PCopyOutMin=[]  PCopyOutMax=[]  NCopyOutDataTypeStr=Inherit: Inherit via back propagation  NCopyOutMin=[]  NCopyOutMax=[]  IntegratorContinuousStateAttributes=''  IntegratorStateMustResolveToSignalObject=off  IntegratorRTWStateStorageClass=Auto  FilterContinuousStateAttributes=''  FilterStateMustResolveToSignalObject=off  FilterRTWStateStorageClass=Auto  ParallelPVariant=Passthrough  IdealPVariant=InternalParameters  IVariant=InternalParameters  DVariant=Disabled  IntegratorVariant=Continuous  SatVariant=Enabled  AWVariant=BackCalculation  PCopyVariant=Disabled  TRVariant=Disabled  FdbkBlocksVariant=Forward  IdealPFdbkVariant=Disabled  SatFdbkVariant=Disabled  DerivativeFilterVariant=Disabled  NVariant=Disabled  NCopyVariant=Disabled_SignalSpec  FilterICVariant=Disabled  IntegratorICVariant=InternalICs  ExternalResetVariant=Disabled  TRSumVariant=Passthrough  SumFdbkVariant=Disabled  SumVariant=Sum_PI  TsampFilterVariant=InternalTs  TsampNgainVariant=Passthrough  TsampIntegralVariant=Disabled_SignalSpec  ExternalSaturationOutDataTypeStr=Inherit: Same as second input
  Product : Product
  Relay : Relay  OnSwitchValue=45  OffSwitchValue=35  OnOutputValue=0  OffOutputValue=1  ZeroCross=off
  Sign : Signum
  Sum : Sum  Inputs=-+|
  Sum1 : Sum  Inputs=-+|
  Switch : Switch  SaturateOnIntegerOverflow=off  InputSameDT=off
  cmd_blower : Outport
  cmd_ptc : Outport  Port=2
  wires:
  T_setpoint/1 -> Sum1/1, Sum/1
  Sum1/1 -> Switch/2, Sign/1
  Product/1 -> PID Controller/1
  PID Controller/1 -> cmd_blower/1
  T_env/1 -> Sum1/2
  Sum/1 -> Product/1
  Sign/1 -> Product/2
  Constant/1 -> Switch/1
  Switch/1 -> cmd_ptc/1
  Relay/1 -> Switch/3
  T_ptc/1 -> Relay/1
  T_cabin/1 -> Sum/2

== system ev_tms_v4_2022/Controls/Compressor Control ==
  p_evap : Inport
  p_chiller : Inport  Port=2
  cmd_chiller_bypass : Inport  Port=3
  ac_onoff : Inport  Port=4
  Constant : Constant
  Constant1 : Constant  Value=0
  Freezing Cutoff : Lookup_n-D  NumberOfTableDimensions=1  BreakpointsForDimension1=[0 0.15 0.25 0.4]  IndexSearchMethod=Linear search  BeginIndexSearchUsingPreviousIndexResult=on  Table=[0 0 1 1]  InternalRulePriority=Speed  RndMeth=Simplest
  MinMax : MinMax  Function=max  Inputs=2  ZeroCross=off
  MinMax1 : MinMax  Inputs=2  ZeroCross=off
  MinMax2 : MinMax  Function=max  Inputs=2
  PID Controller : slpidlib/PID Controller  Controller=PI  Form=Ideal  TimeDomain=Continuous-time  UseExternalTs=off  SampleTime=-1  IntegratorMethod=Forward Euler  FilterMethod=Forward Euler  ControllerParametersSource=internal  P=1  I=1/5  UseKiTs=off  D=0  N=100  UseFilter=on  TunerSelectOption=Transfer Function Based (PID Tuner App)  InitialConditionSource=internal  InitialConditionForIntegrator=0  InitialConditionForFilter=0  DifferentiatorICPrevScaledInput=0  ExternalReset=none  TrackingMode=off  Kt=1  LimitOutput=on  SatLimitsSource=internal  UpperSaturationLimit=1  LowerSaturationLimit=0  LinearizeAsGain=on  AntiWindupMode=back-calculation  Kb=1  LimitIntegrator=off  UpperIntegratorSaturationLimit=inf  LowerIntegratorSaturationLimit=-inf  POutMin=[]  POutMax=[]  IOutMin=[]  IOutMax=[]  DOutMin=[]  DOutMax=[]  NOutMin=[]  NOutMax=[]  SumOutMin=[]  SumOutMax=[]  SaturationOutMin=[]  SaturationOutMax=[]  PParamMin=[]  PParamMax=[]  IParamMin=[]  IParamMax=[]  DParamMin=[]  DParamMax=[]  NParamMin=[]  NParamMax=[]  KbParamMin=[]  KbParamMax=[]  KtParamMin=[]  KtParamMax=[]  KbOutMin=[]  KbOutMax=[]  KtOutMin=[]  KtOutMax=[]  IntegratorOutMin=[]  IntegratorOutMax=[]  FilterOutMin=[]  FilterOutMax=[]  SumI1OutMin=[]  SumI1OutMax=[]  SumI2OutMin=[]  SumI2OutMax=[]  SumI3OutMin=[]  SumI3OutMax=[]  SumI4OutMin=[]  SumI4OutMax=[]  SumDOutMin=[]  SumDOutMax=[]  DifferentiatorOutMin=[]  DifferentiatorOutMax=[]  FilterDiffOutCoefMin=[]  FilterDiffOutCoefMax=[]  ReciprocalOutMin=[]  ReciprocalOutMax=[]  SumDenOutMin=[]  SumDenOutMax=[]  SumNumOutMin=[]  SumNumOutMax=[]  DivideOutMin=[]  DivideOutMax=[]  UdiffTsProdOutMin=[]  UdiffTsProdOutMax=[]  NTsProdOutMin=[]  NTsProdOutMax=[]  UintegralTsProdOutMin=[]  UintegralTsProdOutMax=[]  UngainTsProdOutMin=[]  UngainTsProdOutMax=[]  ClampingZeroOutDataTypeStr=Inherit: Inherit via back propagation  ClampingZeroOutMin=[]  ClampingZeroOutMax=[]  FilterDenConstantOutDataTypeStr=Inherit: Inherit via back propagation  FilterDenConstantOutMin=[]  FilterDenConstantOutMax=[]  PCopyOutDataTypeStr=Inherit: Inherit via back propagation  PCopyOutMin=[]  PCopyOutMax=[]  NCopyOutDataTypeStr=Inherit: Inherit via back propagation  NCopyOutMin=[]  NCopyOutMax=[]  IntegratorContinuousStateAttributes=''  IntegratorStateMustResolveToSignalObject=off  IntegratorRTWStateStorageClass=Auto  FilterContinuousStateAttributes=''  FilterStateMustResolveToSignalObject=off  FilterRTWStateStorageClass=Auto  ParallelPVariant=Passthrough  IdealPVariant=InternalParameters  IVariant=InternalParameters  DVariant=Disabled  IntegratorVariant=Continuous  SatVariant=Enabled  AWVariant=BackCalculation  PCopyVariant=Disabled  TRVariant=Disabled  FdbkBlocksVariant=Forward  IdealPFdbkVariant=Disabled  SatFdbkVariant=Disabled  DerivativeFilterVariant=Disabled  NVariant=Disabled  NCopyVariant=Disabled_SignalSpec  FilterICVariant=Disabled  IntegratorICVariant=InternalICs  ExternalResetVariant=Disabled  TRSumVariant=Passthrough  SumFdbkVariant=Disabled  SumVariant=Sum_PI  TsampFilterVariant=InternalTs  TsampNgainVariant=Passthrough  TsampIntegralVariant=Disabled_SignalSpec  ExternalSaturationOutDataTypeStr=Inherit: Same as second input
  Pressure Target [MPa] : Constant  Value=evaporator_P_target
  Product : Product
  Sum : Sum  Inputs=+-|
  Sum1 : Sum  Inputs=-+|
  Switch : Switch  Criteria=u2 > Threshold  Threshold=0.5  SaturateOnIntegerOverflow=off  InputSameDT=off
  cmd_comp : Outport
  wires:
  cmd_chiller_bypass/1 -> Sum/2
  Constant/1 -> Sum/1
  Sum/1 -> MinMax2/1
  ac_onoff/1 -> MinMax2/2
  Switch/1 -> cmd_comp/1
  Sum1/1 -> PID Controller/1
  MinMax2/1 -> Switch/2
  Product/1 -> Switch/1
  PID Controller/1 -> Product/1
  MinMax1/1 -> Freezing Cutoff/1
  Freezing Cutoff/1 -> Product/2
  p_chiller/1 -> MinMax1/2, MinMax/2
  Constant1/1 -> Switch/3
  Pressure Target [MPa]/1 -> Sum1/1
  p_evap/1 -> MinMax/1, MinMax1/1
  MinMax/1 -> Sum1/2

== system ev_tms_v4_2022/Controls/Coolant Loop Control ==
  T_env : Inport
  T_coolant_battery_in : Inport  Port=2
  T_motor : Inport  Port=3
  T_battery : Inport  Port=4
  T_coolant_inverter_out : Inport  Port=5
  Battery Heater : Subsystem
  Battery Pump : Subsystem
  Chiller Bypass : Subsystem
  Motor Pump : Subsystem
  Parallel-Serial Mode : Subsystem
  Radiator Bypass : Subsystem
  cmd_heater : Outport
  cmd_motor_pump : Outport  Port=2
  cmd_battery_pump : Outport  Port=3
  cmd_chiller_bypass : Outport  Port=4
  cmd_parallel_serial : Outport  Port=5
  cmd_rad_bypass : Outport  Port=6
  wires:
  Parallel-Serial Mode/1(cmd_parallel_serial) -> cmd_parallel_serial/1, Battery Pump/4(parallel_serial)
  Motor Pump/1(cmd_motor_pump) -> Battery Pump/1(cmd_motor_pump), cmd_motor_pump/1
  T_env/1 -> Battery Heater/1(T_env), Parallel-Serial Mode/2(T_env)
  T_coolant_battery_in/1 -> Battery Heater/2(T_coolant_battery_in)
  T_coolant_inverter_out/1 -> Parallel-Serial Mode/3(T_coolant_inverter_out), Radiator Bypass/1(T_coolant_inverter_out)
  T_motor/1 -> Motor Pump/1(T_motor)
  Battery Heater/1(cmd_heater) -> cmd_heater/1
  Battery Pump/1(cmd_battery_pump) -> cmd_battery_pump/1
  Radiator Bypass/1(cmd_rad_bypass) -> cmd_rad_bypass/1
  Chiller Bypass/1(cmd_chiller_bypass) -> Battery Pump/3(cmd_chiller_bypass), Parallel-Serial Mode/1(cmd_chiller_bypass), cmd_chiller_bypass/1
  T_battery/1 -> Chiller Bypass/1(T_battery), Battery Pump/2(T_battery)

== system ev_tms_v4_2022/Controls/Fan Control ==
  p_cond : Inport
  T_env : Inport  Port=2
  cmd_comp : Inport  Port=3
  T_inverter : Inport  Port=4
  T_motor : Inport  Port=5
  Condenser Requirement : Subsystem
  Constant : Constant  Value=0
  Inverter Requirement : Subsystem
  MinMax : MinMax  Function=max  Inputs=3
  Motor Requirement : Subsystem
  Switch : Switch  Criteria=u2 > Threshold  SaturateOnIntegerOverflow=off  InputSameDT=off
  cmd_fan : Outport
  wires:
  MinMax/1 -> cmd_fan/1
  T_motor/1 -> Motor Requirement/1(T_motor)
  T_inverter/1 -> Inverter Requirement/1(T_inverter)
  p_cond/1 -> Condenser Requirement/1(p_cond)
  T_env/1 -> Condenser Requirement/2(T_env)
  cmd_comp/1 -> Switch/2
  Condenser Requirement/1(cmd_fan) -> Switch/1
  Constant/1 -> Switch/3
  Inverter Requirement/1(cmd_fan) -> MinMax/2
  Switch/1 -> MinMax/1
  Motor Requirement/1(cmd_fan) -> MinMax/3
